simulink model "automata_learning"  (R2022a)
settings: Solver=FixedStepAuto  StartTime=0.0  StopTime=10.0  FixedStep=0.01  RelTol=1e-3
settings Model: Creator=diego  LastModifiedBy=diego

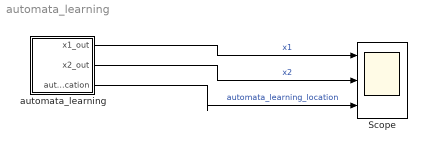
== system automata_learning ==
  Scope : Scope  NumInputPorts=3
  automata_learning : Stateflow chart  TreatAsAtomicUnit=on
  wires:
  automata_learning/1(x1_out) -> Scope/1  "x1"
  automata_learning/2(x2_out) -> Scope/2  "x2"
  automata_learning/3(automata_learning_location) -> Scope/3  "automata_learning_location"

== stateflow chart automata_learning/automata_learning ==
  settings: updateMethod=CONTINUOUS
  state loc1
    du:
    x1_dot = 0.32593727111816406 * (exp(0.48477083444595337 * x1 - 1.148580551147461 * x2 + 0.1389675885438919) - 1.0) / (exp(0.48477083444595337 * x1 - 1.148580551147461 * x2 + 0.1389675885438919) + 1.0) - 0.3596014678478241 * (exp(0.25851118564605713 * x2 - 0.6022998094558716 * x1 + 0.15196284651756287) - 1.0) / (exp(0.25851118564605713 * x2 - 0.6022998094558716 * x1 + 0.15196284651756287) + 1.0) - 0.38119596242904663 * (exp(0.2710812985897064 * x1 + 0.07140150666236877 * x2 - 0.17473101615905762) - 1.0) / (exp(0.2710812985897064 * x1 + 0.07140150666236877 * x2 - 0.17473101615905762) + 1.0) - 0.24526815116405487 * (exp(1.1916418075561523 * x1 + 0.710670530796051 * x2 + 0.14311455190181732) - 1.0) / (exp(1.1916418075561523 * x1 + 0.710670530796051 * x2 + 0.14311455190181732) + 1.0) - 0.5189464092254639 * (exp(0.314195454120636 * x1 + 0.2890457510948181 * x2 + 0.10420307517051697) - 1.0) / (exp(0.314195454120636 * x1 + 0.2890457510948181 * x2 + 0.10420307517051697) + 1.0) - 0.6202051043510437 * (exp(0.5183610320091248 * x2 - 0.7955447435379028 * x1 + 0.18365730345249176) - 1.0) / (exp(0.5183610320091248 * x2 - 0.7955447435379028 * x1 + 0.18365730345249176) + 1.0) - 0.16702140867710114 * (exp(0.6346469521522522 * x1 + 0.09749605506658554 * x2 - 0.16706298291683197) - 1.0) / (exp(0.6346469521522522 * x1 + 0.09749605506658554 * x2 - 0.16706298291683197) + 1.0) - 0.6226367354393005 * (exp(0.07230418920516968 * x1 + 0.731382429599762 * x2 - 0.09759922325611115) - 1.0) / (exp(0.07230418920516968 * x1 + 0.731382429599762 * x2 - 0.09759922325611115) + 1.0) - 0.04186660051345825 * (exp(0.3140783905982971 * x1 + 1.0070087909698486 * x2 - 0.25037726759910583) - 1.0) / (exp(0.3140783905982971 * x1 + 1.0070087909698486 * x2 - 0.25037726759910583) + 1.0) + 0.29658836126327515 * (exp(0.17214448750019073 * x1 + 0.4352760910987854 * x2 + 0.06861189007759094) - 1.0) / (exp(0.17214448750019073 * x1 + 0.4352760910987854 * x2 + 0.06861189007759094) + 1.0) - 0.21561619639396667 * (exp(0.5029935240745544 * x1 + 0.23283125460147858 * x2 - 0.09192439913749695) - 1.0) / (exp(0.5029935240745544 * x1 + 0.23283125460147858 * x2 - 0.09192439913749695) + 1.0) - 0.3064931631088257 * (exp(0.2877821624279022 * x1 - 0.11630978435277939 * x2 + 0.17073462903499603) - 1.0) / (exp(0.2877821624279022 * x1 - 0.11630978435277939 * x2 + 0.17073462903499603) + 1.0) - 0.557625949382782 * (exp(1.022582769393921 * x1 + 0.819436252117157 * x2 + 0.11005283147096634) - 1.0) / (exp(1.022582769393921 * x1 + 0.819436252117157 * x2 + 0.11005283147096634) + 1.0) - 0.010819611139595509 * (exp(0.14163538813591003 * x2 - 0.0128555279225111 * x1 + 0.21235597133636475) - 1.0) / (exp(0.14163538813591003 * x2 - 0.0128555279225111 * x1 + 0.21235597133636475) + 1.0) - 0.11096836626529694 * (exp(0.7596473693847656 * x1 + 0.1486327350139618 * x2 - 0.12276776134967804) - 1.0) / (exp(0.7596473693847656 * x1 + 0.1486327350139618 * x2 - 0.12276776134967804) + 1.0) + 0.34579530358314514 * (exp(1.281874656677246 * x1 - 0.007797074969857931 * x2 + 0.08868469297885895) - 1.0) / (exp(1.281874656677246 * x1 - 0.007797074969857931 * x2 + 0.08868469297885895) + 1.0) + 0.20055410265922546 * (exp(0.6212498545646667 * x1 - 0.47181886434555054 * x2 + 0.20065763592720032) - 1.0) / (exp(0.6212498545646667 * x1 - 0.47181886434555054 * x2 + 0.20065763592720032) + 1.0) + 0.15607209503650665 * (exp(0.5491818189620972 * x1 + 0.932917058467865 * x2 - 0.22964002192020416) - 1.0) / (exp(0.5491818189620972 * x1 + 0.932917058467865 * x2 - 0.22964002192020416) + 1.0) - 0.3019249141216278 * (exp(0.11938861012458801 * x1 + 0.6272786259651184 * x2 - 0.2066216766834259) - 1.0) / (exp(0.11938861012458801 * x1 + 0.6272786259651184 * x2 - 0.2066216766834259) + 1.0) - 0.25567135214805603 * (exp(0.29093700647354126 * x1 + 0.8585092425346375 * x2 + 0.1230396181344986) - 1.0) / (exp(0.29093700647354126 * x1 + 0.8585092425346375 * x2 + 0.1230396181344986) + 1.0) + 0.02639983408153057;
    x2_dot = 0.10304570943117142 * (exp(0.25851118564605713 * x2 - 0.6022998094558716 * x1 + 0.15196284651756287) - 1.0) / (exp(0.25851118564605713 * x2 - 0.6022998094558716 * x1 + 0.15196284651756287) + 1.0) - 0.200416699051857 * (exp(0.3140783905982971 * x1 + 1.0070087909698486 * x2 - 0.25037726759910583) - 1.0) / (exp(0.3140783905982971 * x1 + 1.0070087909698486 * x2 - 0.25037726759910583) + 1.0) - 0.26574644446372986 * (exp(0.2710812985897064 * x1 + 0.07140150666236877 * x2 - 0.17473101615905762) - 1.0) / (exp(0.2710812985897064 * x1 + 0.07140150666236877 * x2 - 0.17473101615905762) + 1.0) + 0.3818143904209137 * (exp(1.1916418075561523 * x1 + 0.710670530796051 * x2 + 0.14311455190181732) - 1.0) / (exp(1.1916418075561523 * x1 + 0.710670530796051 * x2 + 0.14311455190181732) + 1.0) + 0.2950352430343628 * (exp(0.314195454120636 * x1 + 0.2890457510948181 * x2 + 0.10420307517051697) - 1.0) / (exp(0.314195454120636 * x1 + 0.2890457510948181 * x2 + 0.10420307517051697) + 1.0) + 0.38529062271118164 * (exp(0.5183610320091248 * x2 - 0.7955447435379028 * x1 + 0.18365730345249176) - 1.0) / (exp(0.5183610320091248 * x2 - 0.7955447435379028 * x1 + 0.18365730345249176) + 1.0) - 0.17941167950630188 * (exp(0.6346469521522522 * x1 + 0.09749605506658554 * x2 - 0.16706298291683197) - 1.0) / (exp(0.6346469521522522 * x1 + 0.09749605506658554 * x2 - 0.16706298291683197) + 1.0) - 0.031044067814946175 * (exp(0.07230418920516968 * x1 + 0.731382429599762 * x2 - 0.09759922325611115) - 1.0) / (exp(0.07230418920516968 * x1 + 0.731382429599762 * x2 - 0.09759922325611115) + 1.0) + 0.15094634890556335 * (exp(0.48477083444595337 * x1 - 1.148580551147461 * x2 + 0.1389675885438919) - 1.0) / (exp(0.48477083444595337 * x1 - 1.148580551147461 * x2 + 0.1389675885438919) + 1.0) - 0.01213179249316454 * (exp(0.17214448750019073 * x1 + 0.4352760910987854 * x2 + 0.06861189007759094) - 1.0) / (exp(0.17214448750019073 * x1 + 0.4352760910987854 * x2 + 0.06861189007759094) + 1.0) + 0.04754410684108734 * (exp(0.5029935240745544 * x1 + 0.23283125460147858 * x2 - 0.09192439913749695) - 1.0) / (exp(0.5029935240745544 * x1 + 0.23283125460147858 * x2 - 0.09192439913749695) + 1.0) + 0.335369735956192 * (exp(0.2877821624279022 * x1 - 0.11630978435277939 * x2 + 0.17073462903499603) - 1.0) / (exp(0.2877821624279022 * x1 - 0.11630978435277939 * x2 + 0.17073462903499603) + 1.0) + 0.5406773686408997 * (exp(1.022582769393921 * x1 + 0.819436252117157 * x2 + 0.11005283147096634) - 1.0) / (exp(1.022582769393921 * x1 + 0.819436252117157 * x2 + 0.11005283147096634) + 1.0) + 0.4356161653995514 * (exp(0.14163538813591003 * x2 - 0.0128555279225111 * x1 + 0.21235597133636475) - 1.0) / (exp(0.14163538813591003 * x2 - 0.0128555279225111 * x1 + 0.21235597133636475) + 1.0) - 0.00604217778891325 * (exp(0.7596473693847656 * x1 + 0.1486327350139618 * x2 - 0.12276776134967804) - 1.0) / (exp(0.7596473693847656 * x1 + 0.1486327350139618 * x2 - 0.12276776134967804) + 1.0) + 0.28756630420684814 * (exp(1.281874656677246 * x1 - 0.007797074969857931 * x2 + 0.08868469297885895) - 1.0) / (exp(1.281874656677246 * x1 - 0.007797074969857931 * x2 + 0.08868469297885895) + 1.0) + 0.5367230176925659 * (exp(0.6212498545646667 * x1 - 0.47181886434555054 * x2 + 0.20065763592720032) - 1.0) / (exp(0.6212498545646667 * x1 - 0.47181886434555054 * x2 + 0.20065763592720032) + 1.0) - 0.34808170795440674 * (exp(0.5491818189620972 * x1 + 0.932917058467865 * x2 - 0.22964002192020416) - 1.0) / (exp(0.5491818189620972 * x1 + 0.932917058467865 * x2 - 0.22964002192020416) + 1.0) - 0.21330513060092926 * (exp(0.11938861012458801 * x1 + 0.6272786259651184 * x2 - 0.2066216766834259) - 1.0) / (exp(0.11938861012458801 * x1 + 0.6272786259651184 * x2 - 0.2066216766834259) + 1.0) + 0.1417669802904129 * (exp(0.29093700647354126 * x1 + 0.8585092425346375 * x2 + 0.1230396181344986) - 1.0) / (exp(0.29093700647354126 * x1 + 0.8585092425346375 * x2 + 0.1230396181344986) + 1.0) + 0.10780072957277298;
    x1_out=x1;
    x2_out=x2;
    automata_learning_location =1;
  state loc2
    du:
    x1_dot = 0.03149228170514107 * (exp(1.0734007358551025 * x1 + 0.5071157813072205 * x2 - 0.21166552603244781) - 1.0) / (exp(1.0734007358551025 * x1 + 0.5071157813072205 * x2 - 0.21166552603244781) + 1.0) - 0.40203505754470825 * (exp(0.2391774207353592 * x2 - 0.967475414276123 * x1 + 0.1949433535337448) - 1.0) / (exp(0.2391774207353592 * x2 - 0.967475414276123 * x1 + 0.1949433535337448) + 1.0) + 0.02524019405245781 * (exp(0.13369883596897125 * x1 - 0.0795900821685791 * x2 + 0.18307135999202728) - 1.0) / (exp(0.13369883596897125 * x1 - 0.0795900821685791 * x2 + 0.18307135999202728) + 1.0) + 0.2980322241783142 * (exp(0.2512890100479126 * x1 - 0.043760996311903 * x2 + 0.18832963705062866) - 1.0) / (exp(0.2512890100479126 * x1 - 0.043760996311903 * x2 + 0.18832963705062866) + 1.0) - 0.11263395100831985 * (exp(0.1681590974330902 * x1 + 1.1155749559402466 * x2 + 0.19966569542884827) - 1.0) / (exp(0.1681590974330902 * x1 + 1.1155749559402466 * x2 + 0.19966569542884827) + 1.0) - 0.32702845335006714 * (exp(0.633530855178833 * x1 + 0.883022129535675 * x2 - 0.12816235423088074) - 1.0) / (exp(0.633530855178833 * x1 + 0.883022129535675 * x2 - 0.12816235423088074) + 1.0) + 0.26307427883148193 * (exp(0.13530804216861725 * x1 - 0.7477229237556458 * x2 + 0.2005821019411087) - 1.0) / (exp(0.13530804216861725 * x1 - 0.7477229237556458 * x2 + 0.2005821019411087) + 1.0) + 0.5462105870246887 * (exp(0.13939356803894043 * x2 - 0.9821686744689941 * x1 + 0.13904063403606415) - 1.0) / (exp(0.13939356803894043 * x2 - 0.9821686744689941 * x1 + 0.13904063403606415) + 1.0) - 0.11986410617828369 * (exp(0.3031490743160248 * x1 + 0.1992066353559494 * x2 + 0.1736350655555725) - 1.0) / (exp(0.3031490743160248 * x1 + 0.1992066353559494 * x2 + 0.1736350655555725) + 1.0) - 0.393736869096756 * (exp(0.29971739649772644 * x2 - 0.8791264891624451 * x1 + 0.15481750667095184) - 1.0) / (exp(0.29971739649772644 * x2 - 0.8791264891624451 * x1 + 0.15481750667095184) + 1.0) - 0.37582507729530334 * (exp(0.46313202381134033 * x1 + 0.3003675937652588 * x2 - 0.14495442807674408) - 1.0) / (exp(0.46313202381134033 * x1 + 0.3003675937652588 * x2 - 0.14495442807674408) + 1.0) - 0.33854940533638 * (exp(0.5568787455558777 * x1 + 0.9403455257415771 * x2 + 0.17797577381134033) - 1.0) / (exp(0.5568787455558777 * x1 + 0.9403455257415771 * x2 + 0.17797577381134033) + 1.0) - 0.22912773489952087 * (exp(0.09391824156045914 * x2 - 0.6972375512123108 * x1 + 0.012840816751122475) - 1.0) / (exp(0.09391824156045914 * x2 - 0.6972375512123108 * x1 + 0.012840816751122475) + 1.0) - 0.41874393820762634 * (exp(0.5786663293838501 * x2 - 0.9122175574302673 * x1 + 0.1977013200521469) - 1.0) / (exp(0.5786663293838501 * x2 - 0.9122175574302673 * x1 + 0.1977013200521469) + 1.0) - 0.448933482170105 * (exp(0.7480219602584839 * x1 + 0.8157674670219421 * x2 + 0.18014390766620636) - 1.0) / (exp(0.7480219602584839 * x1 + 0.8157674670219421 * x2 + 0.18014390766620636) + 1.0) + 0.06750892847776413 * (exp(0.10911732167005539 * x1 - 0.31921395659446716 * x2 + 0.20562784373760223) - 1.0) / (exp(0.10911732167005539 * x1 - 0.31921395659446716 * x2 + 0.20562784373760223) + 1.0) - 0.0009795943042263389 * (exp(0.643927812576294 * x2 - 0.4227995276451111 * x1 + 0.21201971173286438) - 1.0) / (exp(0.643927812576294 * x2 - 0.4227995276451111 * x1 + 0.21201971173286438) + 1.0) - 0.5558856129646301 * (exp(0.19211773574352264 * x1 + 0.8991435766220093 * x2 + 0.1832033395767212) - 1.0) / (exp(0.19211773574352264 * x1 + 0.8991435766220093 * x2 + 0.1832033395767212) + 1.0) + 0.042215269058942795 * (exp(0.28313499689102173 * x2 - 0.12487761676311493 * x1 + 0.21037372946739197) - 1.0) / (exp(0.28313499689102173 * x2 - 0.12487761676311493 * x1 + 0.21037372946739197) + 1.0) - 0.030157363042235374 * (exp(0.17192572355270386 * x1 + 0.4612632095813751 * x2 - 0.21264176070690155) - 1.0) / (exp(0.17192572355270386 * x1 + 0.4612632095813751 * x2 - 0.21264176070690155) + 1.0) + 0.06722958385944366;
    x2_dot = 0.2109190672636032 * (exp(1.0734007358551025 * x1 + 0.5071157813072205 * x2 - 0.21166552603244781) - 1.0) / (exp(1.0734007358551025 * x1 + 0.5071157813072205 * x2 - 0.21166552603244781) + 1.0) - 0.5727027058601379 * (exp(0.2391774207353592 * x2 - 0.967475414276123 * x1 + 0.1949433535337448) - 1.0) / (exp(0.2391774207353592 * x2 - 0.967475414276123 * x1 + 0.1949433535337448) + 1.0) - 0.08729831129312515 * (exp(0.13369883596897125 * x1 - 0.0795900821685791 * x2 + 0.18307135999202728) - 1.0) / (exp(0.13369883596897125 * x1 - 0.0795900821685791 * x2 + 0.18307135999202728) + 1.0) - 0.19555722177028656 * (exp(0.2512890100479126 * x1 - 0.043760996311903 * x2 + 0.18832963705062866) - 1.0) / (exp(0.2512890100479126 * x1 - 0.043760996311903 * x2 + 0.18832963705062866) + 1.0) - 0.2930713891983032 * (exp(0.1681590974330902 * x1 + 1.1155749559402466 * x2 + 0.19966569542884827) - 1.0) / (exp(0.1681590974330902 * x1 + 1.1155749559402466 * x2 + 0.19966569542884827) + 1.0) + 0.09969780594110489 * (exp(0.633530855178833 * x1 + 0.883022129535675 * x2 - 0.12816235423088074) - 1.0) / (exp(0.633530855178833 * x1 + 0.883022129535675 * x2 - 0.12816235423088074) + 1.0) - 0.31058406829833984 * (exp(0.13530804216861725 * x1 - 0.7477229237556458 * x2 + 0.2005821019411087) - 1.0) / (exp(0.13530804216861725 * x1 - 0.7477229237556458 * x2 + 0.2005821019411087) + 1.0) - 0.023649943992495537 * (exp(0.13939356803894043 * x2 - 0.9821686744689941 * x1 + 0.13904063403606415) - 1.0) / (exp(0.13939356803894043 * x2 - 0.9821686744689941 * x1 + 0.13904063403606415) + 1.0) - 0.07641100138425827 * (exp(0.3031490743160248 * x1 + 0.1992066353559494 * x2 + 0.1736350655555725) - 1.0) / (exp(0.3031490743160248 * x1 + 0.1992066353559494 * x2 + 0.1736350655555725) + 1.0) - 0.3429105877876282 * (exp(0.29971739649772644 * x2 - 0.8791264891624451 * x1 + 0.15481750667095184) - 1.0) / (exp(0.29971739649772644 * x2 - 0.8791264891624451 * x1 + 0.15481750667095184) + 1.0) + 0.0887080505490303 * (exp(0.46313202381134033 * x1 + 0.3003675937652588 * x2 - 0.14495442807674408) - 1.0) / (exp(0.46313202381134033 * x1 + 0.3003675937652588 * x2 - 0.14495442807674408) + 1.0) - 0.18080483376979828 * (exp(0.5568787455558777 * x1 + 0.9403455257415771 * x2 + 0.17797577381134033) - 1.0) / (exp(0.5568787455558777 * x1 + 0.9403455257415771 * x2 + 0.17797577381134033) + 1.0) - 0.12963499128818512 * (exp(0.09391824156045914 * x2 - 0.6972375512123108 * x1 + 0.012840816751122475) - 1.0) / (exp(0.09391824156045914 * x2 - 0.6972375512123108 * x1 + 0.012840816751122475) + 1.0) - 0.5327566862106323 * (exp(0.5786663293838501 * x2 - 0.9122175574302673 * x1 + 0.1977013200521469) - 1.0) / (exp(0.5786663293838501 * x2 - 0.9122175574302673 * x1 + 0.1977013200521469) + 1.0) - 0.21420548856258392 * (exp(0.7480219602584839 * x1 + 0.8157674670219421 * x2 + 0.18014390766620636) - 1.0) / (exp(0.7480219602584839 * x1 + 0.8157674670219421 * x2 + 0.18014390766620636) + 1.0) - 0.3288671672344208 * (exp(0.10911732167005539 * x1 - 0.31921395659446716 * x2 + 0.20562784373760223) - 1.0) / (exp(0.10911732167005539 * x1 - 0.31921395659446716 * x2 + 0.20562784373760223) + 1.0) - 0.30593326687812805 * (exp(0.643927812576294 * x2 - 0.4227995276451111 * x1 + 0.21201971173286438) - 1.0) / (exp(0.643927812576294 * x2 - 0.4227995276451111 * x1 + 0.21201971173286438) + 1.0) - 0.43366116285324097 * (exp(0.19211773574352264 * x1 + 0.8991435766220093 * x2 + 0.1832033395767212) - 1.0) / (exp(0.19211773574352264 * x1 + 0.8991435766220093 * x2 + 0.1832033395767212) + 1.0) - 0.30173683166503906 * (exp(0.28313499689102173 * x2 - 0.12487761676311493 * x1 + 0.21037372946739197) - 1.0) / (exp(0.28313499689102173 * x2 - 0.12487761676311493 * x1 + 0.21037372946739197) + 1.0) + 0.23637011647224426 * (exp(0.17192572355270386 * x1 + 0.4612632095813751 * x2 - 0.21264176070690155) - 1.0) / (exp(0.17192572355270386 * x1 + 0.4612632095813751 * x2 - 0.21264176070690155) + 1.0) - 0.10360264033079147;
    x1_out=x1;
    x2_out=x2;
    automata_learning_location =2;
  loc1 -> loc2 : [0.3288 * x1 - 0.333 * x2 + 1.0 < 0.0]
  (default) -> loc1 : {x1 = 1.0;
      | x2 = -1.0;}
  loc2 -> loc1 : [0.499 * x2 - 0.0006802 * x1 + 1.0 < 0.0]
  data: x1_out output; x1 local; x2_out output; x2 local; automata_learning_location output
  data x1 settings: updateMethod=SF_CONTINUOUS_TIME_DATA
  data x2 settings: updateMethod=SF_CONTINUOUS_TIME_DATA
